simulink model "meart_target_60"  (Simulink 6.5)
settings: Solver=FixedStepDiscrete  StartTime=0.0  StopTime=Inf  FixedStep=0.0005  RelTol=1e-3
values from neighbouring files (symbols this model uses):
  channelmask = ones(1,60)    [run_experiment.m]
  offset = mean(data)    [setthresh.m]
  stimcombs = [I; zeros(60)]    [run_experiment.m]
  stimtimes = (cumsum(dstimtimes)+T_start)*2000    [run_experiment.m]
  stimulusintensity = [400 500 600 700 800]    [run_experiment.m]
  switchtimes = []    [run_experiment.m]
  synctimes = 0    [run_experiment.m]
  threshold = -10*std(data)    [setthresh.m]
undefined symbols (not defined in the file or in its folder): MF, onsetchannelmask, PD2
libraries: simulink x24, meaworklibrary x16, xpclib x9, dspstat3 x2, xpcueilib x2, dspindex x1, dspbuff3 x1, dspsigops x1
(part 1 of 2)
CloseFcn:
  | rtwprivate ssgencode ModelCloseRequest meart_target
settings Model: Creator=cdfz  LastModifiedBy=avnerw  TunableVars=closeonsingleenbale  TunableVarsStorageClass=Auto  BufferReuse=off  ProdHWDeviceType=32-bit xPC Target (AMD Athlon)
settings ConfigSet: SimulationMode=external
settings DataIOCC: LimitDataPoints=off  SignalLogging=off  SaveTime=off
settings OptimizationCC: BlockReduction=off  InlineParams=on  OptimizeBlockIOStorage=off  BufferReuse=off  EnforceIntegerDowncast=off  ExpressionFolding=off  LocalBlockOutputs=off  UseTempVars=on
settings HardwareCC: ProdIntDivRoundTo=Zero  ProdEndianess=LittleEndian  ProdHWDeviceType=32-bit xPC Target (AMD Athlon)
settings RTWCC: SystemTargetFile=xpctarget.tlc  TemplateMakefile=xpc_default_tmf  Description=xPC Target  ProcessScript=xpctarget_make_rtw_hook
settings xpcTargetCC: TargetFcnLib=ansi_tfl_tmw.mat  GenFloatMathFcnCalls=ANSI_C  ExtModeInterfaceLevel=Level2 - Open  RL32LogBufSizeModifier=61*10000*60  RL32IRQSourceModifier=10  xPCIRQSourceBoard=UEI_MFx

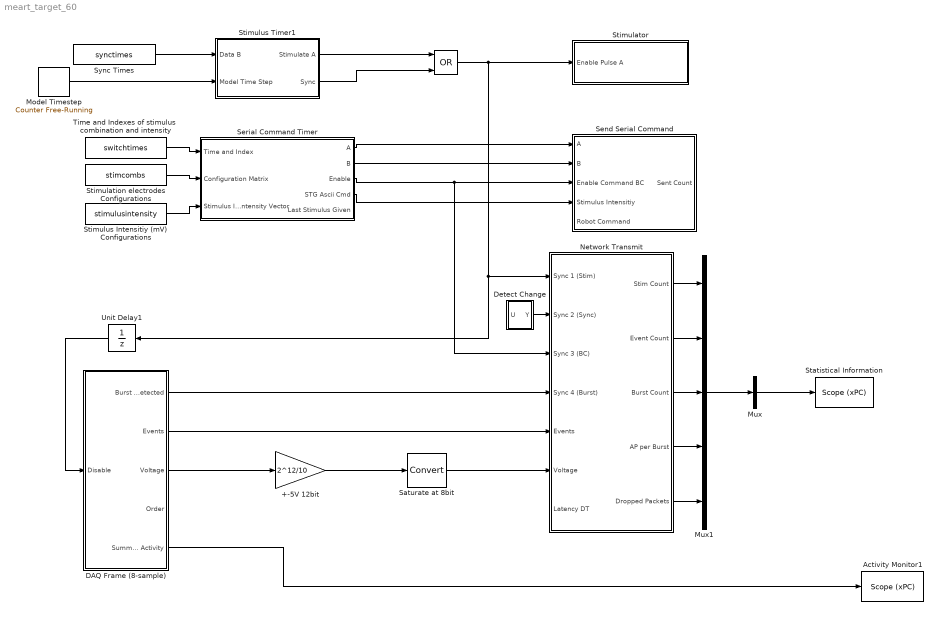
== system meart_target_60 ==
  "      " : Logic  Operator=OR  Inputs=3  IconShape=distinctive  AllPortsSameDT=off  OutDataTypeMode=Boolean
  +-5V 12bit : Gain  Gain=2^12/10  OutDataType=sint(16)  RndMeth=Nearest
  Activity Monitor1 : xpclib/Misc./Scope (xPC)   SystemSampleTime=-1  scopeno=2  scopetype=Target  autostart=on  viewmode=Graphical rolling  formatstr='%15.6f'  grid=on  ylimits=[0,50]  nosamples=500  noprepostsamples=0  interleave=20  triggermode=FreeRun  triggersignal=1  triggerlevel=0.0  triggerslope=Either  triggerscope=1  triggersample=0  filename=data.dat  mode=Lazy  writesize=512  autorestart=off
  DAQ Frame (8-sample) : Subsystem  TreatAsAtomicUnit=on  mask{offset=offset, threshold=threshold, frametime=.0005, refractorytimesamples=6, channelmask=channelmask, blanktimeframes=3, onsetchannelmask=onsetchannelmask, onsetwindowsize=200}
      mask prompts: threshold "Threshold (downward crossing):"; frametime "Frametime (s):"; refractorytimesamples "Refractorytime (frames):"; channelmask "Channelmask (boolean):"; blanktimeframes "Blank time (frames):"; onsetchannelmask "Onset detection channels (logical):"; onsetwindowsize "Onset detection window size (frames)"
  Detect Change : Subsystem  AncestorBlock=|  mask(Detect Change){vinit=0}
      | simulink/Logic and Bit
      | Operations/Detect
      | Change
      mask prompts: vinit "Initial condition:"
      mask help: If the input does not equal its previous value, then output TRUE, otherwise output FALSE. The initial condition determines the initial value of the previous input U/z.
      mask Display: fprintf('U ~= U/z')
  Model Timestep : simulink/Sources/Counter Free-Running  SystemSampleTime=-1  NumBits=32  tsamp=-1
  Mux : Mux  Inputs=1
  Mux1 : Mux  Inputs=5
  "Network Transmit " : Subsystem
  Saturate at 8bit : DataTypeConversion  OutDataTypeMode=int8  RndMeth=Nearest  SaturateOnIntegerOverflow=on
  Send Serial Command : Subsystem
  Serial Command Timer : Subsystem
  Statistical Information : xpclib/Misc./Scope (xPC)   SystemSampleTime=-1  scopeno=4  scopetype=Target  autostart=on  viewmode=Numerical  formatstr="'Stimuli provided    :%13.0f,Events detected     : %15.0f,Bursts detected     : %15.0f,Events per Burst    : %15.0f,UDP Packets Dropped : %15.0f, Delta T:           %15.0f, Clamp Enabled: %15.5f, Clamp Control: %15.0f, Clamp Control2: %15.0f'"  grid=on  ylimits=[0,0]  nosamples=100  noprepostsamples=0  interleave=1  triggermode=FreeRun  triggersignal=1  triggerlevel=0.0  triggerslope=Either  triggerscope=1  triggersample=0  filename=data.dat  mode=Lazy  writesize=512  autorestart=off
  Stimulation electrodes Configurations : Constant  Value=stimcombs  OutDataTypeMode=uint8  OutDataType=sfix(16)  ConRadixGroup=Use specified scaling  OutScaling=2^0  SampleTime=-1  FramePeriod=inf
  Stimulator : Subsystem  TreatAsAtomicUnit=on
  Stimulus Intensitiy (mV) Configurations : Constant  Value=stimulusintensity  OutDataTypeMode=double  OutDataType=sfix(16)  ConRadixGroup=Use specified scaling  OutScaling=2^0  SampleTime=-1  FramePeriod=inf
  Stimulus Timer1 : Subsystem  mask{stimtimes=stimtimes}
      mask prompts: stimtimes "Stimulus Times"
  Sync Times : Constant  Value=synctimes  OutDataTypeMode=uint32  OutDataType=sfix(16)  ConRadixGroup=Use specified scaling  OutScaling=2^0  SampleTime=-1  FramePeriod=inf
  Time and Indexes of stimulus  combination and intensity : Constant  Value=switchtimes  VectorParams1D=off  OutDataTypeMode=uint32  OutDataType=sfix(16)  ConRadixGroup=Use specified scaling  OutScaling=2^0  SampleTime=-1  FramePeriod=inf
  Unit Delay1 : UnitDelay  Orientation=left  SampleTime=-1
  wires:
  DAQ Frame (8-sample)/2(Events) -> "Network Transmit "/5(Events)
  DAQ Frame (8-sample)/3(Voltage) -> +-5V 12bit/1
  +-5V 12bit/1 -> Saturate at 8bit/1
  Mux/1 -> Statistical Information/1
  Saturate at 8bit/1 -> "Network Transmit "/6(Voltage)
  Sync Times/1 -> Stimulus Timer1/1(Data B)
  Serial Command Timer/1(A) -> Send Serial Command/1(A)
  Serial Command Timer/2(B) -> Send Serial Command/2(B)
  Serial Command Timer/3(Enable) -> Send Serial Command/3(Enable Command BC), "Network Transmit "/3(Sync 3 (BC))
  Stimulation electrodes Configurations/1 -> Serial Command Timer/2(Configuration Matrix)
  Time and Indexes of stimulus  combination and intensity/1 -> Serial Command Timer/1(Time and Index)
  DAQ Frame (8-sample)/1(Burst Detected) -> "Network Transmit "/4(Sync 4 (Burst))
  "Network Transmit "/1(Stim Count) -> Mux1/1
  "Network Transmit "/2(Event Count) -> Mux1/2
  "Network Transmit "/3(Burst Count) -> Mux1/3
  "Network Transmit "/4(AP per Burst) -> Mux1/4
  "Network Transmit "/5(Dropped Packets) -> Mux1/5
  Mux1/1 -> Mux/1
  Unit Delay1/1 -> DAQ Frame (8-sample)/1(Disable)
  Stimulus Intensitiy (mV) Configurations/1 -> Serial Command Timer/3(Stimulus Intensity Vector)
  Serial Command Timer/4(STG Ascii Cmd) -> Send Serial Command/4(Stimulus Intensitiy)
  DAQ Frame (8-sample)/5(Summed Activity) -> Activity Monitor1/1
  "      "/1 -> Stimulator/1(Enable Pulse A), "Network Transmit "/1("Sync 1 (Stim)\t"), Unit Delay1/1
  Stimulus Timer1/1(Stimulate A) -> "      "/1
  Stimulus Timer1/2(Sync) -> "      "/3
  Detect Change/1(Y) -> "Network Transmit "/2(Sync 2 (Sync))
  Model Timestep/1 -> Stimulus Timer1/2(Model Time Step)

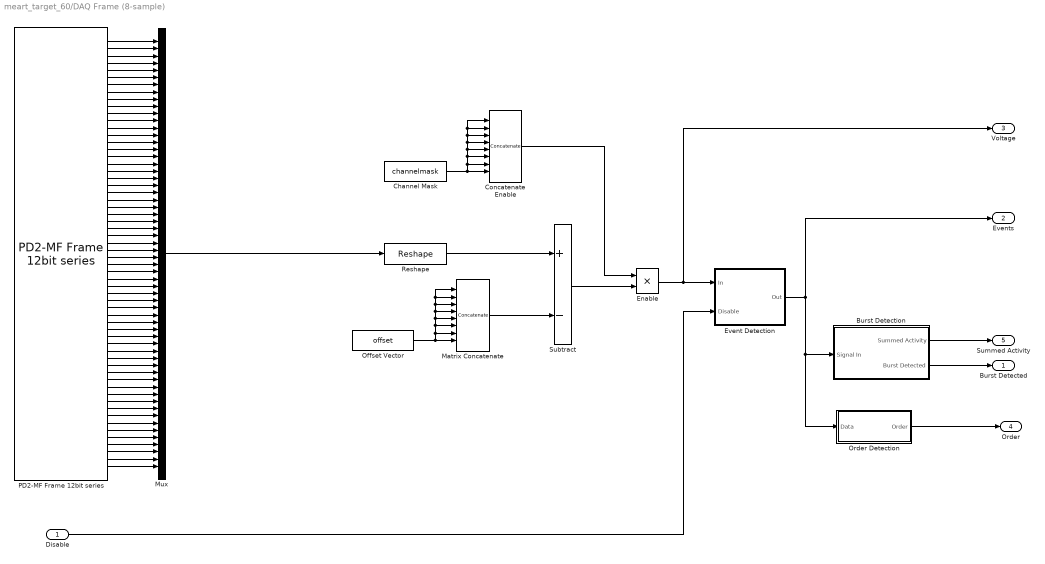
== system meart_target_60/DAQ Frame (8-sample) ==
  Disable : Inport
  Burst Detection : Subsystem  mask{eventrefractorysamples=6, windowsize=0.025, burstthreshold=20, burstrefractorytime=1, sampletime=.0005}
      mask prompts: eventrefractorysamples "Event refractory period (samples):"; windowsize "Spike rate sliding window bin size (s):"; burstthreshold "Burst detection threshold:"; burstrefractorytime "Burst detection refractory period (s):"; sampletime "Sampletime (s)"
      mask Display:
      | plot([.1 .2 .3 .4 .5 .6 .8 .9], [.2 .2 .3 .7 .8 .5 .25 .2])
      | plot([.2 .4], [.3 .3])
      | text(0.1, 0.35, 'th')
  Channel Mask : Constant  Value=channelmask  VectorParams1D=off  OutDataTypeMode=double  OutDataType=sfix(16)  ConRadixGroup=Use specified scaling  OutScaling=2^0  SampleTime=frametime  FramePeriod=inf
  Concatenate Enable : Concatenate  NumInputs=8  Mode=Vertical matrix concatenation
  Enable : Product  Inputs=**  OutScaling=2^-10
  Event Detection : Subsystem
  Matrix Concatenate : Concatenate  NumInputs=8  Mode=Vertical matrix concatenation
  Mux : Mux  Inputs=60
  Offset Vector : Constant  Value=offset  VectorParams1D=off  OutDataTypeMode=double  OutDataType=sfix(16)  ConRadixGroup=Use specified scaling  OutScaling=2^0  SampleTime=frametime  FramePeriod=inf
  Order Detection : Subsystem  mask{buffersizeframes=onsetwindowsize, enablechannelmask=onsetchannelmask}
      mask prompts: buffersizeframes "Buffersize (frames)"; enablechannelmask "Channels to consider (logical):"
  "PD2-MF Frame 12bit series " : xpcueilib/A//D Frame/PD2-MF Frame 12bit series   boardtypein=PD2-MF-64-3M/12H  channel=[1:60]  gain=[1]  mux=[1]  range=+- 5 Volts  sediff=Single Ended  framesize=8  outfmt=Vector  clsource=Internal  scantime=-1  frametime=frametime  sampletime=off  slave=off  freq=8/frametime*60  burst=32  pcislot=-1
  Reshape : Reshape  OutputDimensionality=Customize (N-D)  OutputDimensions=[8,60]
  Subtract : Sum  Inputs=+-  OutScaling=2^-10
  Burst Detected : Outport
  Events : Outport  Port=2
  Voltage : Outport  Port=3
  Order : Outport  Port=4
  Summed Activity : Outport  Port=5
  wires:
  Event Detection/1(Out) -> Burst Detection/1(Signal In), Order Detection/1(Data), Events/1
  Mux/1 -> Reshape/1
  "PD2-MF Frame 12bit series "/60 -> Mux/60
  "PD2-MF Frame 12bit series "/59 -> Mux/59
  "PD2-MF Frame 12bit series "/58 -> Mux/58
  "PD2-MF Frame 12bit series "/57 -> Mux/57
  "PD2-MF Frame 12bit series "/56 -> Mux/56
  "PD2-MF Frame 12bit series "/55 -> Mux/55
  "PD2-MF Frame 12bit series "/54 -> Mux/54
  "PD2-MF Frame 12bit series "/53 -> Mux/53
  "PD2-MF Frame 12bit series "/52 -> Mux/52
  "PD2-MF Frame 12bit series "/51 -> Mux/51
  "PD2-MF Frame 12bit series "/50 -> Mux/50
  "PD2-MF Frame 12bit series "/49 -> Mux/49
  "PD2-MF Frame 12bit series "/48 -> Mux/48
  "PD2-MF Frame 12bit series "/47 -> Mux/47
  "PD2-MF Frame 12bit series "/46 -> Mux/46
  "PD2-MF Frame 12bit series "/45 -> Mux/45
  "PD2-MF Frame 12bit series "/44 -> Mux/44
  "PD2-MF Frame 12bit series "/43 -> Mux/43
  "PD2-MF Frame 12bit series "/42 -> Mux/42
  "PD2-MF Frame 12bit series "/41 -> Mux/41
  "PD2-MF Frame 12bit series "/40 -> Mux/40
  "PD2-MF Frame 12bit series "/39 -> Mux/39
  "PD2-MF Frame 12bit series "/38 -> Mux/38
  "PD2-MF Frame 12bit series "/37 -> Mux/37
  "PD2-MF Frame 12bit series "/36 -> Mux/36
  "PD2-MF Frame 12bit series "/35 -> Mux/35
  "PD2-MF Frame 12bit series "/34 -> Mux/34
  "PD2-MF Frame 12bit series "/33 -> Mux/33
  "PD2-MF Frame 12bit series "/32 -> Mux/32
  "PD2-MF Frame 12bit series "/31 -> Mux/31
  "PD2-MF Frame 12bit series "/30 -> Mux/30
  "PD2-MF Frame 12bit series "/29 -> Mux/29
  "PD2-MF Frame 12bit series "/28 -> Mux/28
  "PD2-MF Frame 12bit series "/27 -> Mux/27
  "PD2-MF Frame 12bit series "/26 -> Mux/26
  "PD2-MF Frame 12bit series "/25 -> Mux/25
  "PD2-MF Frame 12bit series "/24 -> Mux/24
  "PD2-MF Frame 12bit series "/23 -> Mux/23
  "PD2-MF Frame 12bit series "/22 -> Mux/22
  "PD2-MF Frame 12bit series "/21 -> Mux/21
  "PD2-MF Frame 12bit series "/20 -> Mux/20
  "PD2-MF Frame 12bit series "/19 -> Mux/19
  "PD2-MF Frame 12bit series "/18 -> Mux/18
  "PD2-MF Frame 12bit series "/17 -> Mux/17
  "PD2-MF Frame 12bit series "/16 -> Mux/16
  "PD2-MF Frame 12bit series "/15 -> Mux/15
  "PD2-MF Frame 12bit series "/14 -> Mux/14
  "PD2-MF Frame 12bit series "/13 -> Mux/13
  "PD2-MF Frame 12bit series "/12 -> Mux/12
  "PD2-MF Frame 12bit series "/11 -> Mux/11
  "PD2-MF Frame 12bit series "/10 -> Mux/10
  "PD2-MF Frame 12bit series "/9 -> Mux/9
  "PD2-MF Frame 12bit series "/8 -> Mux/8
  "PD2-MF Frame 12bit series "/7 -> Mux/7
  "PD2-MF Frame 12bit series "/6 -> Mux/6
  "PD2-MF Frame 12bit series "/5 -> Mux/5
  "PD2-MF Frame 12bit series "/3 -> Mux/3
  "PD2-MF Frame 12bit series "/4 -> Mux/4
  "PD2-MF Frame 12bit series "/2 -> Mux/2
  "PD2-MF Frame 12bit series "/1 -> Mux/1
  Reshape/1 -> Subtract/1
  Enable/1 -> Voltage/1, Event Detection/1(In)
  Subtract/1 -> Enable/2
  Channel Mask/1 -> Concatenate Enable/8, Concatenate Enable/7, Concatenate Enable/6, Concatenate Enable/5, Concatenate Enable/4, Concatenate Enable/3, Concatenate Enable/2, Concatenate Enable/1
  Concatenate Enable/1 -> Enable/1
  Offset Vector/1 -> Matrix Concatenate/8, Matrix Concatenate/7, Matrix Concatenate/6, Matrix Concatenate/5, Matrix Concatenate/4, Matrix Concatenate/3, Matrix Concatenate/2, Matrix Concatenate/1
  Matrix Concatenate/1 -> Subtract/2
  Order Detection/1(Order) -> Order/1
  Disable/1 -> Event Detection/2(Disable)
  Burst Detection/1(Summed Activity) -> Summed Activity/1
  Burst Detection/2(Burst Detected) -> Burst Detected/1

== system meart_target_60/Detect Change ==
  note: Edge
  note: U(k)
  U : Inport
  Delay Input1 : UnitDelay  Description=Store in Global RAM  X0=vinit  SampleTime=-1
  FixPt Relational Operator : RelationalOperator  Operator=~=  LogicOutDataTypeMode=Boolean  ZeroCross=off
  Y : Outport  InitialOutput=0
  wires:
  FixPt Relational Operator/1 -> Y/1
  Delay Input1/1 -> FixPt Relational Operator/2  "U(k-1)"
  U/1 -> FixPt Relational Operator/1, Delay Input1/1

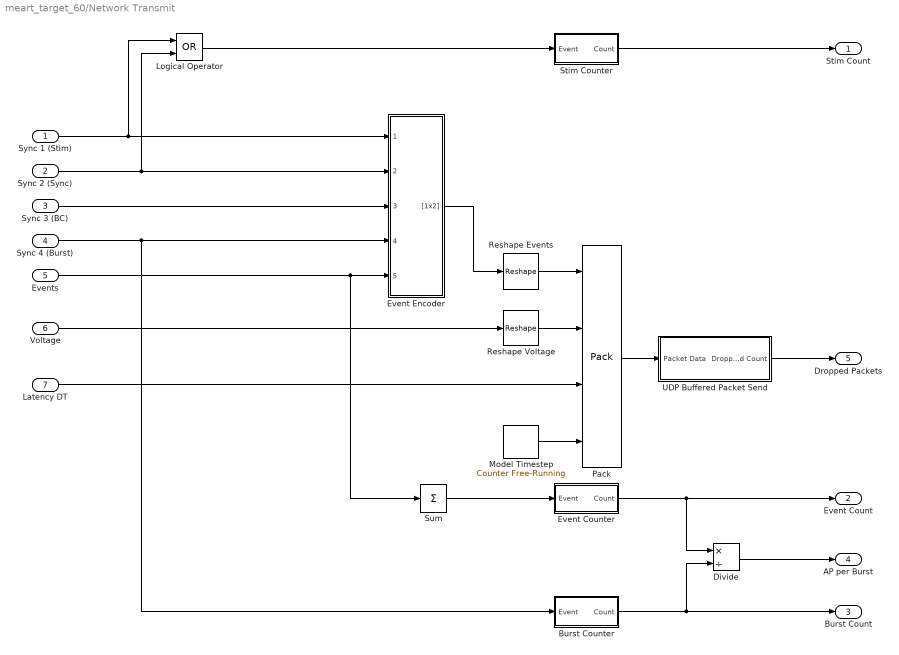
== system meart_target_60/Network Transmit  ==
  "Sync 1 (Stim)\t" : Inport  PortDimensions=1  DataType=boolean
  Sync 2 (Sync) : Inport  Port=2  PortDimensions=1  DataType=boolean
  Sync 3 (BC) : Inport  Port=3  PortDimensions=1  DataType=boolean
  Sync 4 (Burst) : Inport  Port=4  PortDimensions=1  DataType=boolean
  Events : Inport  Port=5  PortDimensions=60  DataType=boolean
  Voltage : Inport  Port=6
  Latency DT : Inport  Port=7  PortDimensions=60  DataType=uint8
  Burst Counter : Subsystem  mask{startvalue=0}
      mask prompts: startvalue "Starting value"
  Divide : Product  Inputs=*/  OutScaling=2^-10
  Event Counter : Subsystem  mask{startvalue=0}
      mask prompts: startvalue "Starting value"
  Event Encoder : Subsystem
  Logical Operator : Logic  Operator=OR  AllPortsSameDT=off  OutDataTypeMode=Boolean
  Model Timestep : simulink/Sources/Counter Free-Running  SystemSampleTime=-1  NumBits=32  tsamp=-1
  Pack : xpclib/UDP/Pack  datatypes={'uint32', 'int8', 'uint8', 'uint32'}  byteAlign=1
  Reshape Events : Reshape
  Reshape Voltage : Reshape
  Stim Counter : Subsystem  mask{startvalue=0}
      mask prompts: startvalue "Starting value"
  Sum : Sum  Inputs=+  OutDataTypeMode=double  OutScaling=2^-10
  UDP Buffered Packet Send : Subsystem
  Stim Count : Outport
  Event Count : Outport  Port=2
  Burst Count : Outport  Port=3
  AP per Burst : Outport  Port=4
  Dropped Packets : Outport  Port=5
  wires:
  Pack/1 -> UDP Buffered Packet Send/1(Packet Data)
  Reshape Voltage/1 -> Pack/2
  UDP Buffered Packet Send/1(Dropped Count) -> Dropped Packets/1
  Voltage/1 -> Reshape Voltage/1
  "Sync 1 (Stim)\t"/1 -> Event Encoder/1(Sync 1), Logical Operator/1
  Sync 4 (Burst)/1 -> Burst Counter/1(Event), Event Encoder/4(Sync 4)
  Sync 3 (BC)/1 -> Event Encoder/3(Sync 3)
  Sync 2 (Sync)/1 -> Event Encoder/2(Sync 2), Logical Operator/2
  Logical Operator/1 -> Stim Counter/1(Event)
  Event Encoder/1("[1x2]") -> Reshape Events/1
  Reshape Events/1 -> Pack/1
  Stim Counter/1(Count) -> Stim Count/1
  Burst Counter/1(Count) -> Burst Count/1, Divide/2
  Event Counter/1(Count) -> Event Count/1, Divide/1
  Events/1 -> Event Encoder/5(Events), Sum/1
  Sum/1 -> Event Counter/1(Event)
  Divide/1 -> AP per Burst/1
  Model Timestep/1 -> Pack/4
  Latency DT/1 -> Pack/3

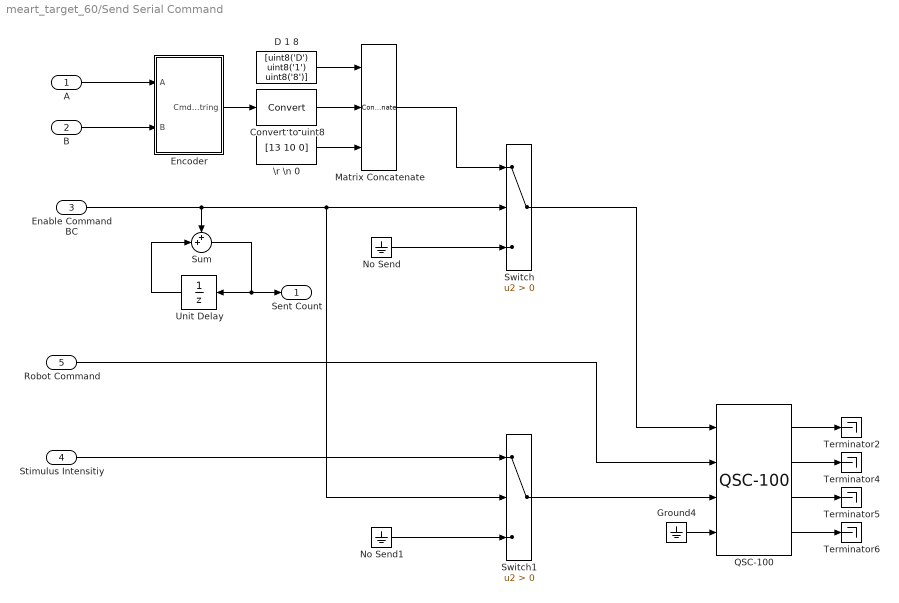
== system meart_target_60/Send Serial Command ==
  A : Inport
  B : Inport  Port=2
  Enable Command BC : Inport  Port=3
  Stimulus Intensitiy : Inport  Port=4
  Robot Command : Inport  Port=5
  Convert to uint8 : DataTypeConversion
  D 1 8 : Constant  Value=[uint8('D') uint8('1') uint8('8')]  OutDataTypeMode=uint8  OutDataType=sfix(16)  ConRadixGroup=Use specified scaling  OutScaling=2^0  SampleTime=inf  FramePeriod=inf
  Encoder : Subsystem
  Ground4 : Ground
  Matrix Concatenate : Concatenate  NumInputs=3  Mode=Vector concatenation
  No Send : Ground
  No Send1 : Ground
  QSC-100 : xpclib/RS232/Quatech/QSC-100/QSC-100  SystemSampleTime=-1  group=Basic Setup  port=3  irqnum=11  slot=-1  baud1=57600  parity1=None  ndata1=8  nstop1=1  fifomode1=16 deep  rlevel1=half full  automode1=off  xmtfifosize1=128  xmtdatatype1=8 bit uint null terminated  rcvfifosize1=128  rcvmaxread1=10  rcvminread1=1  rcvusedelim1=on  rcvdelim1=10  rcvdatatype1=8 bit uint null terminated  rcvsampletime1=0.0005  baud2=9600  parity2=None  ndata2=8  nstop2=1  fifomode2=16 deep  rlevel2=half full  automode2=off  xmtfifosize2=128  xmtdatatype2=count+16 bit uint  rcvfifosize2=128  rcvmaxread2=10  rcvminread2=1  rcvusedelim2=on  rcvdelim2=10  rcvdatatype2=8 bit uint null terminated  rcvsampletime2=0.0005  baud3=115200  parity3=None  ndata3=8  nstop3=1  fifomode3=16 deep  rlevel3=half full  automode3=off  xmtfifosize3=128  xmtdatatype3=8 bit uint null terminated  rcvfifosize3=128  rcvmaxread3=1024  rcvminread3=1  rcvusedelim3=on  rcvdelim3=13  rcvdatatype3=count+16 bit uint  rcvsampletime3=0.0005  buad4=115200  parity4=None  ndata4=8  nstop4=1  fifomode4=64 deep  rlevel4=half full  automode4=on  xmtfifosize4=1024  xmtdatatype4=8 bit uint null terminated  rcvfifosize4=1024  rcvmaxread4=1024  rcvminread4=1  rcvusedelim4=on  rcvdelim4=13  rcvdatatype4=count+16 bit uint  rcvsampletime4=0.0005
  Sum : Sum  Inputs=++|  OutDataTypeMode=double
  Switch : Switch  Criteria=u2 > Threshold  ZeroCross=off
  Switch1 : Switch  Criteria=u2 > Threshold  ZeroCross=off
  Terminator{2,4..6} (4 alike) : Terminator
  Unit Delay : UnitDelay  Orientation=left  SampleTime=-1
  \r \n 0 : Constant  Value=[13 10 0]  OutDataTypeMode=uint8  OutDataType=sfix(16)  ConRadixGroup=Use specified scaling  OutScaling=2^0  SampleTime=inf  FramePeriod=inf
  Sent Count : Outport
  wires:
  Encoder/1(CmdString) -> Convert to uint8/1
  Convert to uint8/1 -> Matrix Concatenate/2
  \r \n 0/1 -> Matrix Concatenate/3
  D 1 8/1 -> Matrix Concatenate/1
  A/1 -> Encoder/1(A)
  B/1 -> Encoder/2(B)
  Enable Command BC/1 -> Sum/1, Switch/2, Switch1/2
  No Send/1 -> Switch/3
  Matrix Concatenate/1 -> Switch/1
  Switch/1 -> QSC-100/1
  Sum/1 -> Unit Delay/1, Sent Count/1
  Unit Delay/1 -> Sum/2
  QSC-100/1 -> Terminator2/1
  QSC-100/2 -> Terminator4/1
  QSC-100/3 -> Terminator5/1
  QSC-100/4 -> Terminator6/1
  Ground4/1 -> QSC-100/4
  Robot Command/1 -> QSC-100/2
  No Send1/1 -> Switch1/3
  Switch1/1 -> QSC-100/3
  Stimulus Intensitiy/1 -> Switch1/1

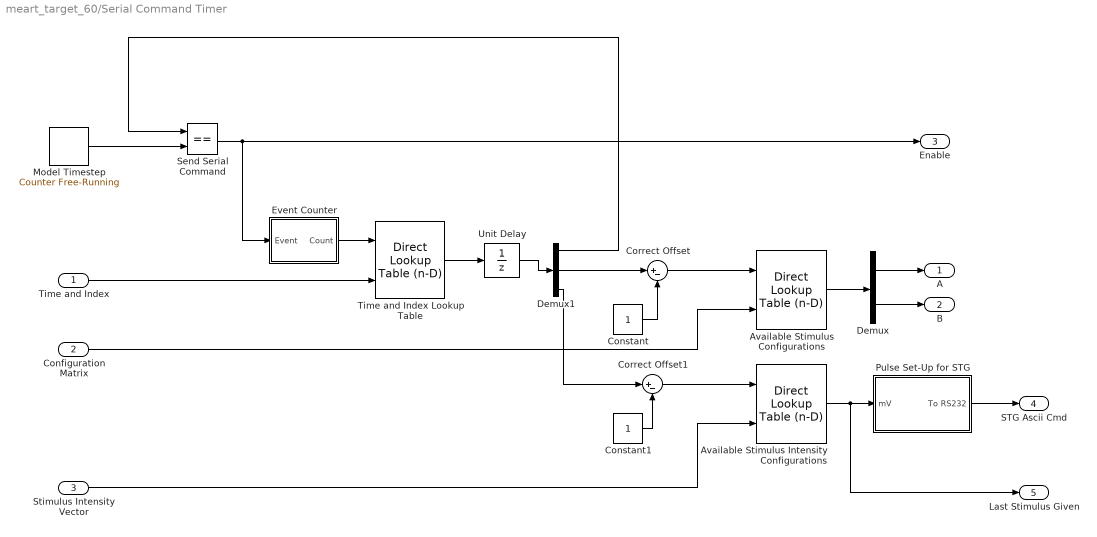
== system meart_target_60/Serial Command Timer ==
  Time and Index : Inport  DataType=uint32
  Configuration Matrix : Inport  Port=2  DataType=uint8
  Stimulus Intensity Vector : Inport  Port=3  DataType=double
  Available Stimulus Configurations : simulink/Lookup Tables/Direct Lookup Table (n-D)  maskTabDims=2  explicitNumDims=1  outDims=Column  tabIsInput=on  mxTable=[eye(60); eye(60)]  clipFlag=Warning
  Available Stimulus Intensity Configurations : simulink/Lookup Tables/Direct Lookup Table (n-D)  maskTabDims=1  explicitNumDims=1  outDims=Element  tabIsInput=on  mxTable=[eye(60); eye(60)]  clipFlag=Warning
  Constant : Constant  Value=1  OutDataType=sfix(16)  ConRadixGroup=Use specified scaling  OutScaling=2^0  SampleTime=inf  FramePeriod=inf
  Constant1 : Constant  Value=1  OutDataType=sfix(16)  ConRadixGroup=Use specified scaling  OutScaling=2^0  SampleTime=inf  FramePeriod=inf
  Correct Offset : Sum  Inputs=|+-
  Correct Offset1 : Sum  Inputs=|+-
  Demux : Demux  Outputs=2
  Demux1 : Demux  Outputs=3
  Event Counter : Subsystem  mask{startvalue=0}
      mask prompts: startvalue "Starting value"
  Model Timestep : simulink/Sources/Counter Free-Running  SystemSampleTime=-1  NumBits=32  tsamp=-1
  Pulse Set-Up for STG : Subsystem
  Send Serial Command : RelationalOperator  Operator===  LogicOutDataTypeMode=Boolean  LogicDataType=uint(32)  InputSameDT=on
  Time and Index Lookup Table : simulink/Lookup Tables/Direct Lookup Table (n-D)  maskTabDims=2  explicitNumDims=1  outDims=Column  tabIsInput=on  mxTable="[1250:1250:125000000;  repmat(59:-1:50,1,10000)]"  clipFlag=Warning
  Unit Delay : UnitDelay  SampleTime=-1
  A : Outport
  B : Outport  Port=2
  Enable : Outport  Port=3
  STG Ascii Cmd : Outport  Port=4
  Last Stimulus Given : Outport  Port=5
  wires:
  Demux/2 -> B/1
  Demux/1 -> A/1
  Time and Index Lookup Table/1 -> Unit Delay/1
  Demux1/1 -> Send Serial Command/1
  Available Stimulus Configurations/1 -> Demux/1
  Send Serial Command/1 -> Enable/1, Event Counter/1(Event)
  Event Counter/1(Count) -> Time and Index Lookup Table/1
  Configuration Matrix/1 -> Available Stimulus Configurations/2
  Time and Index/1 -> Time and Index Lookup Table/2
  Model Timestep/1 -> Send Serial Command/2
  Demux1/2 -> Correct Offset/1
  Correct Offset/1 -> Available Stimulus Configurations/1
  Constant/1 -> Correct Offset/2
  Unit Delay/1 -> Demux1/1
  Demux1/3 -> Correct Offset1/1
  Constant1/1 -> Correct Offset1/2
  Correct Offset1/1 -> Available Stimulus Intensity Configurations/1
  Stimulus Intensity Vector/1 -> Available Stimulus Intensity Configurations/2
  Available Stimulus Intensity Configurations/1 -> Pulse Set-Up for STG/1(mV), Last Stimulus Given/1
  Pulse Set-Up for STG/1(To RS232) -> STG Ascii Cmd/1

== system meart_target_60/Stimulator ==
  Enable Pulse A : Inport  DataType=boolean
  Blanking Signal A : Subsystem  mask{dilation=2}
      mask Display:
      | plot([.1 .2 .2 .3 .4 .4 .5], [.1 .1 .9 .9 .9 .1 .1])
      | plot([.5 .8 .8 .9], [.9 .9 .1 .1])
      | plot([.5 .7 .65 .7 .65], [.3 .3 .35 .3 .25])
      | text(0.5, 0.6, num2str(dilation))
  Data Type Conversion A : DataTypeConversion  OutDataTypeMode=double
  PD2-MF 12bit series : xpcueilib/Digital Output/PD2-MF 12bit series  boardtypein=PD2-MF-64-3M/12H  channel=[1 2]  reset=[1]  initValue=[0]  sampletime=-1  pcislot=-1
  wires:
  Enable Pulse A/1 -> Data Type Conversion A/1
  Blanking Signal A/1(Out) -> PD2-MF 12bit series/2
  Data Type Conversion A/1 -> PD2-MF 12bit series/1, Blanking Signal A/1(In)

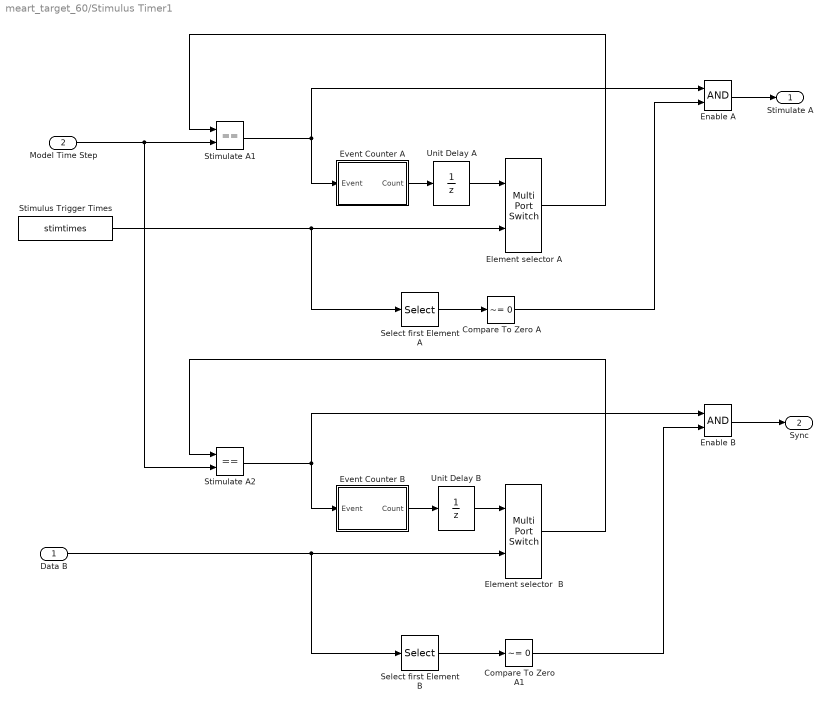
== system meart_target_60/Stimulus Timer1 ==
  Data B : Inport
  Model Time Step : Inport  Port=2  DataType=uint32
  Compare To Zero A : simulink/Logic and Bit Operations/Compare To Zero  SystemSampleTime=-1  relop=~=  LogicOutDataTypeMode=boolean  ZeroCross=off
  Compare To Zero A1 : simulink/Logic and Bit Operations/Compare To Zero  SystemSampleTime=-1  relop=~=  LogicOutDataTypeMode=boolean  ZeroCross=off
  Element selector  B : MultiPortSwitch  Inputs=1  zeroidx=on
  Element selector A : MultiPortSwitch  Inputs=1  zeroidx=on
  Enable A : Logic  AllPortsSameDT=off  OutDataTypeMode=Boolean
  Enable B : Logic  AllPortsSameDT=off  OutDataTypeMode=Boolean
  Event Counter A : Subsystem  mask{startvalue=0}
      mask prompts: startvalue "Starting value"
  Event Counter B : Subsystem  mask{startvalue=0}
      mask prompts: startvalue "Starting value"
  Select first Element A : Selector  InputType=Vector  ElementSrc=Internal  Elements=1  RowSrc=Internal  Rows=1  ColumnSrc=Internal  Columns=1  IndexIsStartValue=off
  Select first Element B : Selector  InputType=Vector  ElementSrc=Internal  Elements=1  RowSrc=Internal  Rows=1  ColumnSrc=Internal  Columns=1  IndexIsStartValue=off
  Stimulate A1 : RelationalOperator  Operator===  LogicOutDataTypeMode=Boolean  LogicDataType=uint(32)  ZeroCross=off
  Stimulate A2 : RelationalOperator  Operator===  LogicOutDataTypeMode=Boolean  LogicDataType=uint(32)  ZeroCross=off
  Stimulus Trigger Times : Constant  Value=stimtimes  OutDataTypeMode=uint32  OutDataType=sfix(16)  ConRadixGroup=Use specified scaling  OutScaling=2^0  SampleTime=-1  FramePeriod=inf
  Unit Delay A : UnitDelay  SampleTime=-1
  Unit Delay B : UnitDelay  SampleTime=-1
  Stimulate A : Outport
  Sync : Outport  Port=2
  wires:
  Select first Element B/1 -> Compare To Zero A1/1
  Select first Element A/1 -> Compare To Zero A/1
  Compare To Zero A1/1 -> Enable B/2
  Enable B/1 -> Sync/1
  Compare To Zero A/1 -> Enable A/2
  Enable A/1 -> Stimulate A/1
  Unit Delay B/1 -> Element selector  B/1
  Unit Delay A/1 -> Element selector A/1
  Element selector  B/1 -> Stimulate A2/1
  Data B/1 -> Select first Element B/1, Element selector  B/2
  Event Counter B/1(Count) -> Unit Delay B/1
  Stimulate A2/1 -> Enable B/1, Event Counter B/1(Event)
  Element selector A/1 -> Stimulate A1/1
  Stimulus Trigger Times/1 -> Select first Element A/1, Element selector A/2
  Event Counter A/1(Count) -> Unit Delay A/1
  Model Time Step/1 -> Stimulate A2/2, Stimulate A1/2
  Stimulate A1/1 -> Enable A/1, Event Counter A/1(Event)

== system meart_target_60/DAQ Frame (8-sample)/Burst Detection ==
  Signal In : Inport
  Burst Refractory : Subsystem  mask{refractorysamples=round(burstrefractorytime/sampletime)}
      mask prompts: refractorysamples "Refractory time (samples)"
      mask Display:
      | plot([.1 .2 .2 .2 .4 .4 .4 .6 .6 .6 .8 .8 .8 .9], [.1 .1 .9 .1 .1 .4 .1 .1 .4 .1 .1 .9 .1 .1])
      | plot([.35 .45], [.4 .4])
      | plot([.55 .65], [.4 .4])
      | text(0.35, 0.6, num2str(refractorysamples))
  Constant : Constant  Value=burstthreshold  OutDataTypeMode=double  OutDataType=sfix(16)  ConRadixGroup=Use specified scaling  OutScaling=2^0  SampleTime=-1  FramePeriod=inf
  Data Type Conversion : DataTypeConversion
  Dilate : Subsystem  mask{dilation=round(windowsize/sampletime)}
      mask Display:
      | plot([.1 .2 .2 .3 .3 .4 .4 .5], [.1 .1 .6 .6 .9 .9 .1 .1])
      | plot([.5 .8 .8 .9], [.9 .9 .1 .1])
      | plot([.5 .7 .65 .7 .65], [.3 .3 .35 .3 .25])
      | text(0.5, 0.6, num2str(dilation))
  Event Refractory : Subsystem  mask{refractorysamples=eventrefractorysamples}
      mask prompts: refractorysamples "Refractory period (samples):"
      mask Display:
      | plot([.1 .3 .3 .3 .5 .5 .5 .7 .7 .7 .9], [.1 .1 .9 .1 .1 .4 .1 .1 .9 .1 .1])
      | plot([.4 .6], [.4 .4])
      | text(0.45, 0.6, num2str(refractorysamples))
  Relational Operator : RelationalOperator  Operator=>  LogicOutDataTypeMode=Boolean  ZeroCross=off
  Sumate : Sum  Inputs=+  OutScaling=2^-10
  Summed Activity : Outport
  Burst Detected : Outport  Port=2
  wires:
  Dilate/1(Out) -> Summed Activity/1, Relational Operator/1
  Relational Operator/1 -> Burst Refractory/1(Signal In)
  Constant/1 -> Relational Operator/2
  Burst Refractory/1(Signal Out) -> Burst Detected/1
  Sumate/1 -> Dilate/1(In)
  Event Refractory/1(Out1) -> Data Type Conversion/1
  Data Type Conversion/1 -> Sumate/1
  Signal In/1 -> Event Refractory/1(In1)

== system meart_target_60/DAQ Frame (8-sample)/Event Detection ==
  In : Inport
  Disable : Inport  Port=2
  Detect Spike Time : Subsystem  TreatAsAtomicUnit=on
      mask Display:
      | plot([.1 .44 .48 .52 .56 .9], [.5 .5 .9 .1 .5 .5])
      | plot([.4 .65], [.3 .3])
      | text(0.3, 0.35, 'th')
  Held Disable : Subsystem  mask{disabletimesamples=blanktimeframes}
      mask prompts: disabletimesamples "Number of samples to hold disable for:"
  Hit  Crossing : HitCross  HitCrossingOffset=threshold  HitCrossingDirection=falling
  Minimum : dspstat3/Minimum  DialogController=dspfixptddg.MinMax  DialogControllerArgs=DataTag0  fcn=Value  reset=None  indexBase=One  operateOver=Each column  colComp=on  operation=minimum  roundingMode=Floor  overflowMode=off
  Refractory : Subsystem  mask{refractoryperiod=refractorytimesamples}
      mask prompts: refractoryperiod "Refractory period (samples):"
      mask Display:
      | plot([.1 .3 .3 .3 .5 .5 .5 .7 .7 .7 .9], [.1 .1 .9 .1 .1 .4 .1 .1 .9 .1 .1])
      | plot([.4 .6], [.4 .4])
      | text(0.4, 0.6, num2str(refractoryperiod))
  Out : Outport
  wires:
  Minimum/1 -> Hit  Crossing/1
  Hit  Crossing/1 -> Refractory/1(In1)
  In/1 -> Minimum/1
  Held Disable/1(Out) -> Out/1
  Disable/1 -> Held Disable/1(Disable)
  Refractory/1(Out1) -> Held Disable/2(Signal)

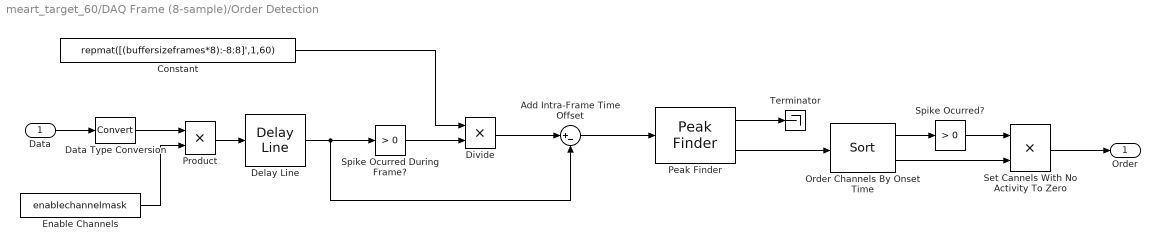
== system meart_target_60/DAQ Frame (8-sample)/Order Detection ==
  Data : Inport
  Add Intra-Frame Time Offset : Sum  Inputs=|+-  OutDataTypeMode=uint32
  Constant : Constant  Value=repmat([(buffersizeframes*8):-8:8]',1,60)  VectorParams1D=off  OutDataTypeMode=uint32  OutDataType=sfix(16)  ConRadixGroup=Use specified scaling  OutScaling=2^0  SampleTime=inf  FramePeriod=inf
  Data Type Conversion : DataTypeConversion  OutDataTypeMode=int8
  Delay Line : dspbuff3/Delay Line  siz=buffersizeframes  ic=0  directfeed=off
  Divide : Product  Inputs=**  OutDataTypeMode=uint32  OutScaling=2^-10
  Enable Channels : Constant  Value=enablechannelmask  OutDataTypeMode=int8  OutDataType=sfix(16)  ConRadixGroup=Use specified scaling  OutScaling=2^0  SampleTime=inf  FramePeriod=inf
  Order Channels By Onset Time : dspstat3/Sort  DialogController=dspDDGCreate  DialogControllerArgs=DataTag1  otype=Value and Index  dir=Descending  sortAlg=Insertion sort  roundingMode=Floor  overflowMode=off
  Peak Finder : dspsigops/Peak Finder  DialogController=dspdialog.PeakFinder  DialogControllerArgs=DataTag2  polarity=Maxima  outputIdx=off  outputVal=on  maxPeaks=1  NoiseDistinguish=off  thresh=0  roundingMode=Floor  overflowMode=off
      settings: allowOverrides=off
  Product : Product  OutDataTypeMode=int8  RndMeth=Zero
  Set Cannels With No Activity To Zero : Product  OutDataTypeMode=uint8  RndMeth=Zero
  Spike Ocurred During Frame? : simulink/Logic and Bit Operations/Compare To Zero  SystemSampleTime=-1  relop=>  LogicOutDataTypeMode=boolean  ZeroCross=off
  Spike Ocurred? : simulink/Logic and Bit Operations/Compare To Zero  SystemSampleTime=-1  relop=>  LogicOutDataTypeMode=uint8  ZeroCross=off
  Terminator : Terminator
  Order : Outport
  wires:
  Delay Line/1 -> Spike Ocurred During Frame?/1, Add Intra-Frame Time Offset/2
  Order Channels By Onset Time/1 -> Spike Ocurred?/1
  Spike Ocurred?/1 -> Set Cannels With No Activity To Zero/1
  Order Channels By Onset Time/2 -> Set Cannels With No Activity To Zero/2
  Peak Finder/2 -> Order Channels By Onset Time/1
  Peak Finder/1 -> Terminator/1
  Add Intra-Frame Time Offset/1 -> Peak Finder/1
  Set Cannels With No Activity To Zero/1 -> Order/1
  Spike Ocurred During Frame?/1 -> Divide/2
  Divide/1 -> Add Intra-Frame Time Offset/1
  Constant/1 -> Divide/1
  Data/1 -> Data Type Conversion/1
  Data Type Conversion/1 -> Product/1
  Product/1 -> Delay Line/1
  Enable Channels/1 -> Product/2

== system meart_target_60/Network Transmit /Burst Counter ==
  Event : Inport
  Sum : Sum  Inputs=|++  OutDataTypeMode=double
  Unit Delay : UnitDelay  Orientation=left  X0=startvalue  SampleTime=-1
  Count : Outport
  wires:
  Event/1 -> Sum/1
  Sum/1 -> Count/1, Unit Delay/1
  Unit Delay/1 -> Sum/2

== system meart_target_60/Network Transmit /Event Counter ==
  Event : Inport
  Sum : Sum  Inputs=|++  InputSameDT=on
  Unit Delay : UnitDelay  Orientation=left  X0=startvalue  SampleTime=-1
  Count : Outport
  wires:
  Unit Delay/1 -> Sum/2
  Sum/1 -> Unit Delay/1, Count/1
  Event/1 -> Sum/1

== system meart_target_60/Network Transmit /Event Encoder ==
  Sync 1 : Inport  PortDimensions=1  DataType=boolean
  Sync 2 : Inport  Port=2  PortDimensions=1  DataType=boolean
  Sync 3 : Inport  Port=3  PortDimensions=1
  Sync 4 : Inport  Port=4  PortDimensions=1  DataType=boolean
  Events : Inport  Port=5  PortDimensions=[1 60]  DataType=boolean
  Data Type Conversion : DataTypeConversion  OutDataTypeMode=uint32  RndMeth=Simplest
  Encode Matrix : Constant  Value=[1 0; 2 0; 2^2 0; 2^3 0; 2^4 0; 2^5 0; 2^6 0; 2^7 0; 2^8 0; 2^9 0; 2^10 0; 2^11 0; 2^12 0; 2^13 0; 2^14 0; 2^15 0; 2^16 0; 2^17 0; 2^18 0; 2^19 0; 2^20 0; 2^21 0; 2^22 0; 2^23 0; 2^24 0; 2^25 0; 2^26 0; 2^27 0; 2^28 0; 2^29 0; 2^30 0; 2^31 0; 0 1; 0 2; 0 2^2; 0 2^3; 0 2^4; 0 2^5; 0 2^6; 0 2^7; 0 2^8; 0 2^9; 0 2^10; 0 2^11; 0 2^12; 0 2^13; 0 2^14; 0 2^15; 0 2^16; 0 2^17; 0 2^18; 0 2^19; 0 2^20; 0 2^21; 0 2^22; 0 2^23; 0 2^24; 0 2^25; 0 2^26; 0 2^27; 0 2^28; 0 2^29; 0 2^30; 0 2^31]  OutDataTypeMode=uint32  OutDataType=sfix(16)  ConRadixGroup=Use specified scaling  OutScaling=2^0  SampleTime=inf  FramePeriod=inf
  Matrix Concatenation : Concatenate  NumInputs=5  Mode=Vector concatenation
  Product : Product  Multiplication=Matrix(*)  OutDataTypeMode=uint32  RndMeth=Simplest  InputSameDT=on
  Reshape : Reshape  OutputDimensionality=Row vector (2-D)
  "[1x2]" : Outport
  wires:
  Encode Matrix/1 -> Product/2
  Data Type Conversion/1 -> Product/1
  Product/1 -> "[1x2]"/1
  Reshape/1 -> Matrix Concatenation/1
  Events/1 -> Reshape/1
  Sync 1/1 -> Matrix Concatenation/2
  Sync 2/1 -> Matrix Concatenation/3
  Sync 3/1 -> Matrix Concatenation/4
  Sync 4/1 -> Matrix Concatenation/5
  Matrix Concatenation/1 -> Data Type Conversion/1

== system meart_target_60/Network Transmit /Stim Counter ==
  Event : Inport
  Sum : Sum  Inputs=|++  OutDataTypeMode=double
  Unit Delay : UnitDelay  Orientation=left  X0=startvalue  SampleTime=-1
  Count : Outport
  wires:
  Unit Delay/1 -> Sum/2
  Sum/1 -> Unit Delay/1, Count/1
  Event/1 -> Sum/1

== system meart_target_60/Network Transmit /UDP Buffered Packet Send ==
  Packet Data : Inport
  Acknowledge : xpclib/UDP/Receive  ipAddress=192.168.0.1  ipPort=25001  width=4  sampletime=-1
  Data Packet Transmission : Subsystem  TreatAsAtomicUnit=on
  Data packet fifo : S-Function  FunctionName=xpcregstack  Parameters=psize,bsize  mask{psize=10, bsize=1000}
      mask prompts: psize "Packet Size"; bsize "Packet Buffers"
      mask Display:
      | port_label('output',1,'q')
      | port_label('output',2,'valid')
      | port_label('output',3,'drop')
      | port_label('input',1,'d')
      | port_label('input',2,'ack')
  Transmit Logic : Stateflow chart
  Unit Delay : UnitDelay  Orientation=left  SampleTime=-1
  Unpack : xpclib/UDP/Unpack  dimensions={[1]}  datatypes={'uint32'}  byteAlign=1
  Width1 : Width  Orientation=up
  Dropped Count : Outport
  wires:
  Acknowledge/1 -> Unpack/1
  Unpack/1 -> Transmit Logic/1(rcv_sync)
  Acknowledge/2 -> Transmit Logic/2(rcv_valid)
  Data packet fifo/1 -> Width1/1, Data Packet Transmission/2(Data)
  Data packet fifo/2 -> Transmit Logic/4(dv)
  Unit Delay/1 -> Data packet fifo/2
  Data packet fifo/3 -> Dropped Count/1
  Width1/1 -> Transmit Logic/3(packsize)
  Transmit Logic/3(ack) -> Unit Delay/1
  Transmit Logic/2(send_sync) -> Data Packet Transmission/1(Sync)
  Transmit Logic/1(send_packet) -> Data Packet Transmission/Enable
  Packet Data/1 -> Data packet fifo/1

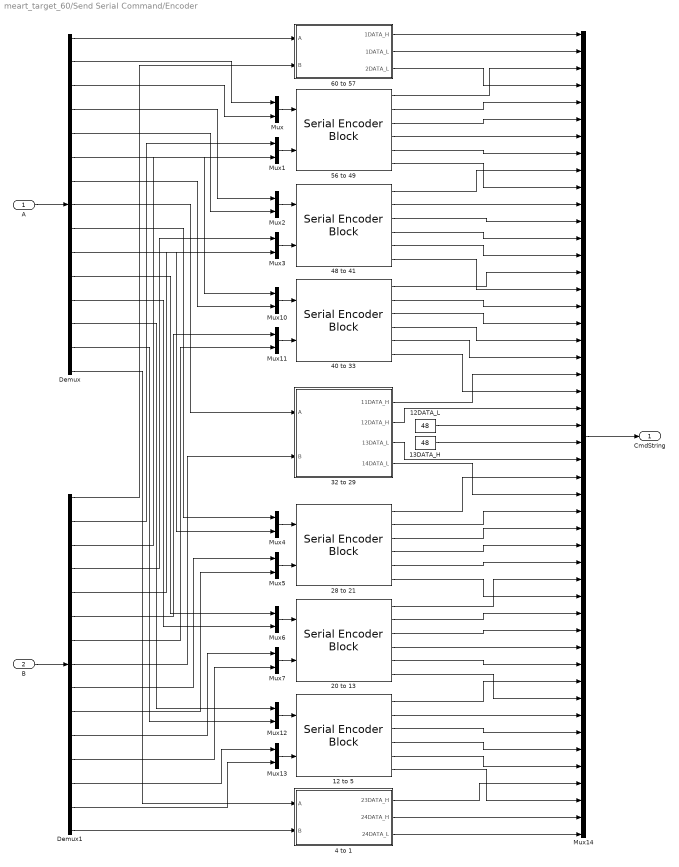
== system meart_target_60/Send Serial Command/Encoder ==
  A : Inport  PortDimensions=60
  B : Inport  Port=2  PortDimensions=60
  12 to 5 : meaworklibrary/Serial Encoder Block  SystemSampleTime=-1
  12DATA_L : Constant  Value=48  OutDataTypeMode=uint8  OutDataType=sfix(16)  ConRadixGroup=Use specified scaling  OutScaling=2^0  SampleTime=inf  FramePeriod=inf
  13DATA_H : Constant  Value=48  OutDataTypeMode=uint8  OutDataType=sfix(16)  ConRadixGroup=Use specified scaling  OutScaling=2^0  SampleTime=inf  FramePeriod=inf
  20 to 13 : meaworklibrary/Serial Encoder Block  SystemSampleTime=-1
  28 to 21 : meaworklibrary/Serial Encoder Block  SystemSampleTime=-1
  32 to 29 : Subsystem
  4 to 1 : Subsystem
  40 to 33 : meaworklibrary/Serial Encoder Block  SystemSampleTime=-1
  48 to 41 : meaworklibrary/Serial Encoder Block  SystemSampleTime=-1
  56 to 49 : meaworklibrary/Serial Encoder Block  SystemSampleTime=-1
  60 to 57 : Subsystem
  Demux : Demux  Outputs=15
  Demux1 : Demux  Outputs=15
  Mux{,1..7,10..13} (12 alike) : Mux  Inputs=2
  Mux14 : Mux  Inputs=48
  CmdString : Outport
  wires:
  A/1 -> Demux/1
  B/1 -> Demux1/1
  Mux/1 -> 56 to 49/1
  Mux1/1 -> 56 to 49/2
  Mux2/1 -> 48 to 41/1
  Mux3/1 -> 48 to 41/2
  Mux4/1 -> 28 to 21/1
  Mux5/1 -> 28 to 21/2
  Mux6/1 -> 20 to 13/1
  Mux7/1 -> 20 to 13/2
  Mux10/1 -> 40 to 33/1
  Mux11/1 -> 40 to 33/2
  Mux12/1 -> 12 to 5/1
  Mux13/1 -> 12 to 5/2
  Demux/1 -> 60 to 57/1(A)
  Demux/2 -> Mux/1
  Demux/3 -> Mux/2
  Demux/4 -> Mux2/1
  Demux/5 -> Mux2/2
  Demux/6 -> Mux10/1
  Demux/7 -> Mux10/2
  Demux1/1 -> 60 to 57/2(B)
  Demux1/2 -> Mux1/1
  Demux1/3 -> Mux1/2
  Demux1/4 -> Mux3/1
  Demux1/5 -> Mux3/2
  Demux1/6 -> Mux11/1
  Demux1/7 -> Mux11/2
  60 to 57/1(1DATA_H) -> Mux14/1
  4 to 1/3(24DATA_L) -> Mux14/48
  4 to 1/2(24DATA_H) -> Mux14/47
  60 to 57/2(1DATA_L) -> Mux14/2
  Demux1/15 -> 4 to 1/2(B)
  Demux/8 -> 32 to 29/1(A)
  Demux/9 -> Mux4/1
  Demux/10 -> Mux4/2
  Demux/11 -> Mux6/1
  Demux/12 -> Mux6/2
  Demux/13 -> Mux12/1
  Demux/14 -> Mux12/2
  Demux/15 -> 4 to 1/1(A)
  Demux1/8 -> 32 to 29/2(B)
  Demux1/9 -> Mux5/1
  Demux1/10 -> Mux5/2
  Demux1/11 -> Mux7/1
  Demux1/12 -> Mux7/2
  Demux1/13 -> Mux13/1
  Demux1/14 -> Mux13/2
  60 to 57/3(2DATA_L) -> Mux14/4
  56 to 49/1 -> Mux14/3
  56 to 49/2 -> Mux14/5
  56 to 49/3 -> Mux14/6
  56 to 49/4 -> Mux14/7
  56 to 49/6 -> Mux14/10
  48 to 41/1 -> Mux14/9
  48 to 41/2 -> Mux14/11
  48 to 41/4 -> Mux14/13
  48 to 41/5 -> Mux14/14
  48 to 41/6 -> Mux14/16
  40 to 33/1 -> Mux14/15
  40 to 33/2 -> Mux14/17
  40 to 33/3 -> Mux14/18
  40 to 33/4 -> Mux14/19
  40 to 33/5 -> Mux14/20
  40 to 33/6 -> Mux14/22
  32 to 29/1(11DATA_H) -> Mux14/21
  12DATA_L/1 -> Mux14/24
  13DATA_H/1 -> Mux14/25
  32 to 29/2(12DATA_H) -> Mux14/23
  32 to 29/3(13DATA_L) -> Mux14/26
  32 to 29/4(14DATA_L) -> Mux14/28
  28 to 21/1 -> Mux14/27
  28 to 21/2 -> Mux14/29
  28 to 21/3 -> Mux14/30
  28 to 21/4 -> Mux14/31
  28 to 21/5 -> Mux14/32
  28 to 21/6 -> Mux14/34
  20 to 13/1 -> Mux14/33
  20 to 13/2 -> Mux14/35
  20 to 13/3 -> Mux14/36
  20 to 13/4 -> Mux14/37
  20 to 13/5 -> Mux14/38
  20 to 13/6 -> Mux14/40
  12 to 5/1 -> Mux14/39
  12 to 5/2 -> Mux14/41
  12 to 5/3 -> Mux14/42
  12 to 5/4 -> Mux14/43
  12 to 5/5 -> Mux14/44
  12 to 5/6 -> Mux14/46
  4 to 1/1(23DATA_H) -> Mux14/45
  Mux14/1 -> CmdString/1
  56 to 49/5 -> Mux14/8
  48 to 41/3 -> Mux14/12

== system meart_target_60/Serial Command Timer/Event Counter ==
  Event : Inport
  Data Type Conversion : DataTypeConversion  OutDataTypeMode=uint8
  Sum : Sum  Inputs=|++  OutDataTypeMode=uint32
  Unit Delay : UnitDelay  Orientation=left  X0=startvalue  SampleTime=-1
  Count : Outport
  wires:
  Unit Delay/1 -> Sum/2
  Sum/1 -> Unit Delay/1, Count/1
  Event/1 -> Data Type Conversion/1
  Data Type Conversion/1 -> Sum/1

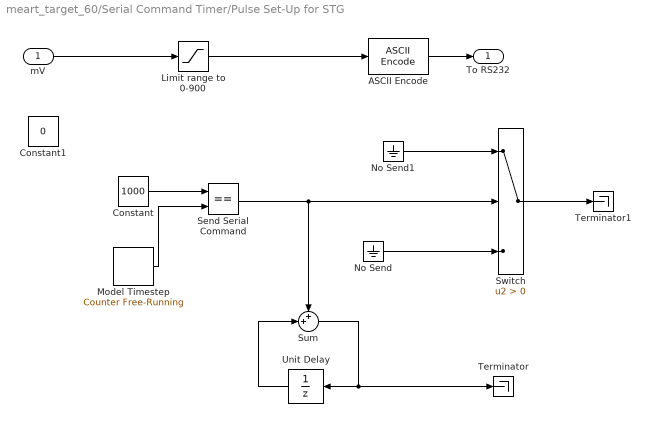
== system meart_target_60/Serial Command Timer/Pulse Set-Up for STG ==
  mV : Inport
  "ASCII Encode " : xpclib/RS232/ASCII Encode   format=prog k1;ranges=3;pulses=1;-%04i;wait1=2;pulses=1;0;\r\n  nvars=1  maxlength=128  vartypes={ 'double' }
  Constant : Constant  Value=1000  OutDataTypeMode=uint32  OutDataType=sfix(16)  ConRadixGroup=Use specified scaling  OutScaling=2^0  SampleTime=inf  FramePeriod=inf
  Constant1 : Constant  Value=0  OutDataTypeMode=double  OutDataType=sfix(16)  ConRadixGroup=Use specified scaling  OutScaling=2^0  SampleTime=inf  FramePeriod=inf
  Limit range to 0-900 : Saturate  UpperLimit=900  LowerLimit=0
  Model Timestep : simulink/Sources/Counter Free-Running  SystemSampleTime=-1  NumBits=32  tsamp=-1
  No Send : Ground
  No Send1 : Ground
  Send Serial Command : RelationalOperator  Operator===  LogicOutDataTypeMode=Boolean  LogicDataType=uint(32)  InputSameDT=on
  Sum : Sum  Inputs=++|  OutDataTypeMode=double
  Switch : Switch  Criteria=u2 > Threshold  ZeroCross=off
  Terminator : Terminator
  Terminator1 : Terminator
  Unit Delay : UnitDelay  Orientation=left  SampleTime=-1
  To RS232 : Outport
  wires:
  mV/1 -> Limit range to 0-900/1
  Model Timestep/1 -> Send Serial Command/2
  Constant/1 -> Send Serial Command/1
  Send Serial Command/1 -> Switch/2, Sum/1
  Switch/1 -> Terminator1/1
  Sum/1 -> Unit Delay/1, Terminator/1
  Unit Delay/1 -> Sum/2
  Limit range to 0-900/1 -> "ASCII Encode "/1
  No Send/1 -> Switch/3
  "ASCII Encode "/1 -> To RS232/1
  No Send1/1 -> Switch/1

== system meart_target_60/Stimulator/Blanking Signal A ==
  In : Inport
  Add : Sum  Inputs=++-  OutScaling=2^-10
  Integer Delay : simulink/Discrete/Integer Delay  vinit=0.0  samptime=-1  NumDelays=1
  Integer Delay1 : simulink/Discrete/Integer Delay  vinit=0.0  samptime=-1  NumDelays=dilation
  Out : Outport
  wires:
  Add/1 -> Integer Delay/1, Out/1
  Integer Delay1/1 -> Add/3
  Integer Delay/1 -> Add/1
  In/1 -> Add/2, Integer Delay1/1

== system meart_target_60/Stimulus Timer1/Event Counter A ==
  Event : Inport
  Data Type Conversion : DataTypeConversion  OutDataTypeMode=uint32
  Sum : Sum  Inputs=|++
  Unit Delay : UnitDelay  Orientation=left  X0=startvalue  SampleTime=-1
  Count : Outport
  wires:
  Data Type Conversion/1 -> Sum/1
  Event/1 -> Data Type Conversion/1
  Sum/1 -> Count/1, Unit Delay/1
  Unit Delay/1 -> Sum/2

== system meart_target_60/Stimulus Timer1/Event Counter B ==
  Event : Inport
  Data Type Conversion : DataTypeConversion  OutDataTypeMode=uint32
  Sum : Sum  Inputs=|++
  Unit Delay : UnitDelay  Orientation=left  X0=startvalue  SampleTime=-1
  Count : Outport
  wires:
  Unit Delay/1 -> Sum/2
  Sum/1 -> Unit Delay/1, Count/1
  Event/1 -> Data Type Conversion/1
  Data Type Conversion/1 -> Sum/1

== system meart_target_60/DAQ Frame (8-sample)/Burst Detection/Burst Refractory ==
  Signal In : Inport  DataType=boolean
  Logical Operator : Logic  AllPortsSameDT=off  OutDataTypeMode=Boolean
  Triggered Disable : Subsystem  mask{holdtimesamples=refractorysamples}
      mask prompts: holdtimesamples "Hold time (samples)"
      mask Display:
      | plot([.1 .2 .2 .2 .3], [.5  .5 .9 .5 .5 ])
      | plot([.3 .8 .8 .9], [.1 .1 .5 .5])
      | plot([.3 .7 .65 .7 .65], [.65 .65 .70 .65 .60])
      | text(0.4, 0.35, num2str(holdtimesamples))
  Unit Delay : UnitDelay  SampleTime=-1
  Signal Out : Outport
  wires:
  Signal In/1 -> Unit Delay/1, Logical Operator/2
  Unit Delay/1 -> Triggered Disable/1(Trigger)
  Logical Operator/1 -> Signal Out/1
  Triggered Disable/1(Enable) -> Logical Operator/1

== system meart_target_60/DAQ Frame (8-sample)/Burst Detection/Dilate ==
  In : Inport
  Add : Sum  Inputs=++-  OutScaling=2^-10
  Dilate Delay : simulink/Discrete/Integer Delay  vinit=0.0  samptime=-1  NumDelays=dilation
  Loop Delay : simulink/Discrete/Integer Delay  vinit=0.0  samptime=-1  NumDelays=1
  Out : Outport
  wires:
  In/1 -> Dilate Delay/1, Add/2
  Loop Delay/1 -> Add/1
  Dilate Delay/1 -> Add/3
  Add/1 -> Out/1, Loop Delay/1

== system meart_target_60/DAQ Frame (8-sample)/Burst Detection/Event Refractory ==
  In1 : Inport
  Integer Delay1 : simulink/Discrete/Integer Delay  Orientation=left  vinit=0  samptime=-1  NumDelays=1
  Logical Operator : Logic  AllPortsSameDT=off  OutDataTypeMode=Boolean
  Loop : simulink/Discrete/Integer Delay  Orientation=left  vinit=1  samptime=-1  NumDelays=1
  Re-Enable : simulink/Discrete/Integer Delay  Orientation=left  vinit=0  samptime=-1  NumDelays=refractorysamples
  addition-modulo-two : Logic  Orientation=left  Operator=XOR  Inputs=3  AllPortsSameDT=off  OutDataTypeMode=Boolean
  Out1 : Outport
  wires:
  Re-Enable/1 -> addition-modulo-two/3
  Loop/1 -> addition-modulo-two/1
  Integer Delay1/1 -> addition-modulo-two/2
  addition-modulo-two/1 -> Logical Operator/1, Loop/1
  Logical Operator/1 -> Re-Enable/1, Integer Delay1/1, Out1/1
  In1/1 -> Logical Operator/2

== system meart_target_60/DAQ Frame (8-sample)/Event Detection/Detect Spike Time ==
  Signal : Inport
  Current below : RelationalOperator  Operator=<  LogicOutDataTypeMode=Boolean
  For Iterator : ForIterator  IterationLimit=8  IterationVariableDataType=int8
  Ground : Ground
  Logical Operator : Logic  AllPortsSameDT=off  OutDataTypeMode=Boolean
  Previous above : RelationalOperator  LogicOutDataTypeMode=Boolean
  Switch : Switch  Criteria=u2 ~= 0
  Threshold : Constant  Value=threshold  OutDataType=sfix(16)  ConRadixGroup=Use specified scaling  OutScaling=2^0  SampleTime=inf  FramePeriod=inf
  Unit Delay : UnitDelay  X0=-100  SampleTime=-1
  Variable Selector : dspindex/Variable Selector  NumInputs=1  rowsOrCols=Rows  IdxMode=Variable  Elements=[1 3]  ZerOneIdxMode=One-based  errmode=Generate Error  FillMode=off  FillValues=0
  Out : Outport  DataType=int8
  wires:
  Threshold/1 -> Previous above/1, Current below/2
  Unit Delay/1 -> Previous above/2
  Current below/1 -> Logical Operator/1
  Previous above/1 -> Logical Operator/2
  Signal/1 -> Variable Selector/1
  Variable Selector/1 -> Current below/1, Unit Delay/1
  For Iterator/1 -> Switch/1, Variable Selector/2
  Switch/1 -> Out/1
  Logical Operator/1 -> Switch/2
  Ground/1 -> Switch/3

== system meart_target_60/DAQ Frame (8-sample)/Event Detection/Held Disable ==
  Disable : Inport  DataType=boolean
  Signal : Inport  Port=2
  Ground : Ground
  Logical Operator : Logic  Operator=OR  Inputs=1  AllPortsSameDT=off  OutDataTypeMode=Boolean
  Switch : Switch  Criteria=u2 ~= 0  ZeroCross=off
  Tapped Delay : simulink/Discrete/Tapped Delay  vinit=0.0  samptime=-1  NumDelays=disabletimesamples  DelayOrder=Oldest  includeCurrent=on
  Out : Outport
  wires:
  Switch/1 -> Out/1
  Logical Operator/1 -> Switch/2
  Disable/1 -> Tapped Delay/1
  Ground/1 -> Switch/1
  Signal/1 -> Switch/3
  Tapped Delay/1 -> Logical Operator/1

== system meart_target_60/DAQ Frame (8-sample)/Event Detection/Refractory ==
  In1 : Inport
  Integer Delay1 : simulink/Discrete/Integer Delay  Orientation=left  vinit=0  samptime=-1  NumDelays=1
  Logical Operator : Logic  AllPortsSameDT=off  OutDataTypeMode=Boolean
  Loop : simulink/Discrete/Integer Delay  Orientation=left  vinit=1  samptime=-1  NumDelays=1
  Re-Enable : simulink/Discrete/Integer Delay  Orientation=left  vinit=0  samptime=-1  NumDelays=refractoryperiod
  addition-modulo-two : Logic  Orientation=left  Operator=XOR  Inputs=3  AllPortsSameDT=off  OutDataTypeMode=Boolean
  Out1 : Outport
  wires:
  In1/1 -> Logical Operator/2
  Logical Operator/1 -> Out1/1, Integer Delay1/1, Re-Enable/1
  addition-modulo-two/1 -> Loop/1, Logical Operator/1
  Integer Delay1/1 -> addition-modulo-two/2
  Loop/1 -> addition-modulo-two/1
  Re-Enable/1 -> addition-modulo-two/3

== system meart_target_60/Network Transmit /UDP Buffered Packet Send/Data Packet Transmission ==
  Sync : Inport
  Data : Inport  Port=2
  Enable : EnablePort
  Pack : xpclib/UDP/Pack  datatypes={'uint32','uint8'}  byteAlign=1
  UDP Send : xpclib/UDP/Send  ipAddress=192.168.0.1  ipPort=25000  localPort=-1  sampletime=-1
  wires:
  Data/1 -> Pack/2
  Sync/1 -> Pack/1
  Pack/1 -> UDP Send/1

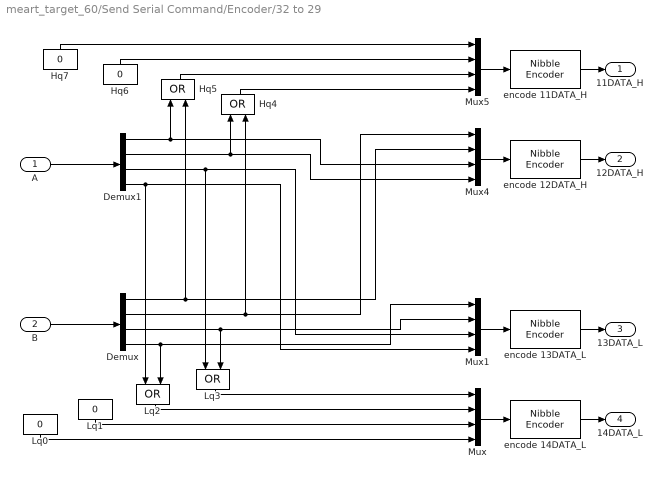
== system meart_target_60/Send Serial Command/Encoder/32 to 29 ==
  A : Inport  PortDimensions=4
  B : Inport  Port=2  PortDimensions=4
  Demux : Demux
  Demux1 : Demux
  Hq4 : Logic  Orientation=up  Operator=OR  AllPortsSameDT=off  OutDataTypeMode=Specify via dialog
  Hq5 : Logic  Orientation=up  Operator=OR  AllPortsSameDT=off  OutDataTypeMode=Specify via dialog
  Hq6 : Constant  Orientation=up  Value=0  OutDataTypeMode=uint8  OutDataType=sfix(16)  ConRadixGroup=Use specified scaling  OutScaling=2^0  SampleTime=inf  FramePeriod=inf
  Hq7 : Constant  Orientation=up  Value=0  OutDataTypeMode=uint8  OutDataType=sfix(16)  ConRadixGroup=Use specified scaling  OutScaling=2^0  SampleTime=inf  FramePeriod=inf
  Lq0 : Constant  Orientation=down  Value=0  OutDataTypeMode=uint8  OutDataType=sfix(16)  ConRadixGroup=Use specified scaling  OutScaling=2^0  SampleTime=inf  FramePeriod=inf
  Lq1 : Constant  Orientation=down  Value=0  OutDataTypeMode=uint8  OutDataType=sfix(16)  ConRadixGroup=Use specified scaling  OutScaling=2^0  SampleTime=inf  FramePeriod=inf
  Lq2 : Logic  Orientation=down  Operator=OR  AllPortsSameDT=off  OutDataTypeMode=Specify via dialog
  Lq3 : Logic  Orientation=down  Operator=OR  AllPortsSameDT=off  OutDataTypeMode=Specify via dialog
  Mux{,1,4..5} (4 alike) : Mux
  encode 11DATA_H : meaworklibrary/Nibble Encoder  SystemSampleTime=-1
  encode 12DATA_H : meaworklibrary/Nibble Encoder  SystemSampleTime=-1
  encode 13DATA_L : meaworklibrary/Nibble Encoder  SystemSampleTime=-1
  encode 14DATA_L : meaworklibrary/Nibble Encoder  SystemSampleTime=-1
  11DATA_H : Outport  DataType=uint8
  12DATA_H : Outport  Port=2  DataType=uint8
  13DATA_L : Outport  Port=3  DataType=uint8
  14DATA_L : Outport  Port=4  DataType=uint8
  wires:
  B/1 -> Demux/1
  A/1 -> Demux1/1
  Mux4/1 -> encode 12DATA_H/1
  encode 12DATA_H/1 -> 12DATA_H/1
  Mux1/1 -> encode 13DATA_L/1
  encode 13DATA_L/1 -> 13DATA_L/1
  Demux1/1 -> Mux4/3, Hq5/1
  Demux/1 -> Mux4/2, Hq5/2
  Demux1/2 -> Mux4/4, Hq4/1
  Demux/2 -> Mux4/1, Hq4/2
  Demux1/3 -> Mux1/3, Lq3/1
  Demux/3 -> Mux1/2, Lq3/2
  Demux1/4 -> Mux1/4, Lq2/1
  Demux/4 -> Mux1/1, Lq2/2
  Mux5/1 -> encode 11DATA_H/1
  encode 11DATA_H/1 -> 11DATA_H/1
  Hq5/1 -> Mux5/3
  Hq4/1 -> Mux5/4
  Hq6/1 -> Mux5/2
  Hq7/1 -> Mux5/1
  Mux/1 -> encode 14DATA_L/1
  encode 14DATA_L/1 -> 14DATA_L/1
  Lq3/1 -> Mux/1
  Lq2/1 -> Mux/2
  Lq1/1 -> Mux/3
  Lq0/1 -> Mux/4

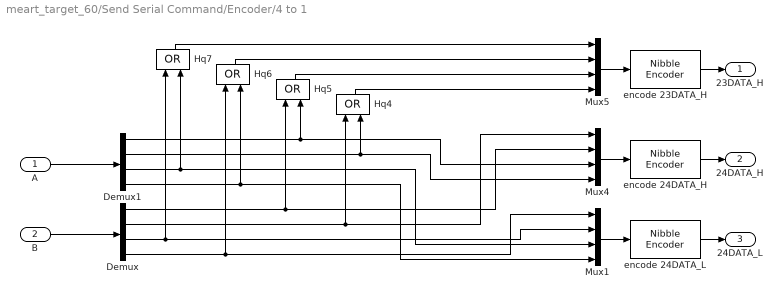
== system meart_target_60/Send Serial Command/Encoder/4 to 1 ==
  A : Inport  PortDimensions=4
  B : Inport  Port=2  PortDimensions=4
  Demux : Demux
  Demux1 : Demux
  Hq{4..7} (4 alike) : Logic  Orientation=up  Operator=OR  AllPortsSameDT=off  OutDataTypeMode=Specify via dialog
  Mux1 : Mux
  Mux4 : Mux
  Mux5 : Mux
  encode 23DATA_H : meaworklibrary/Nibble Encoder  SystemSampleTime=-1
  encode 24DATA_H : meaworklibrary/Nibble Encoder  SystemSampleTime=-1
  encode 24DATA_L : meaworklibrary/Nibble Encoder  SystemSampleTime=-1
  23DATA_H : Outport  DataType=uint8
  24DATA_H : Outport  Port=2  DataType=uint8
  24DATA_L : Outport  Port=3  DataType=uint8
  wires:
  B/1 -> Demux/1
  A/1 -> Demux1/1
  Mux4/1 -> encode 24DATA_H/1
  encode 24DATA_H/1 -> 24DATA_H/1
  Mux1/1 -> encode 24DATA_L/1
  encode 24DATA_L/1 -> 24DATA_L/1
  Demux1/1 -> Mux4/3, Hq5/2
  Demux/1 -> Mux4/2, Hq5/1
  Demux1/2 -> Mux4/4, Hq4/2
  Demux/2 -> Mux4/1, Hq4/1
  Demux1/3 -> Mux1/3, Hq7/2
  Demux/3 -> Mux1/2, Hq7/1
  Demux1/4 -> Mux1/4, Hq6/2
  Demux/4 -> Mux1/1, Hq6/1
  Mux5/1 -> encode 23DATA_H/1
  encode 23DATA_H/1 -> 23DATA_H/1
  Hq5/1 -> Mux5/3
  Hq4/1 -> Mux5/4
  Hq6/1 -> Mux5/2
  Hq7/1 -> Mux5/1
